simulink model "GreenHydrogenMicrogrid"  (R2026a)
settings: Solver=FixedStepAuto  StopTime=24*3600*7.5  FixedStep=Ts  MaxStep=0.1  AbsTol=1e-3
PreLoadFcn:
  | GreenHydrogenMicrogridData;
undefined symbols (not defined in the file): Battery, DiscIntNeverNeededParam, Electrolyzer, Operation_Ref, Plate, R_h2, Tank, Ts
libraries: fl_lib x35, nesl_utility x15, ee_lib x4, simulink x3, batteryecm_lib x1
(part 3 of 3)

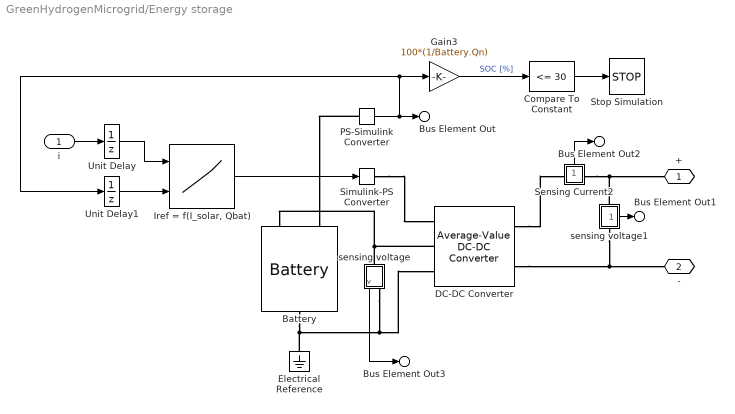
== system GreenHydrogenMicrogrid/Energy storage ==
  i : Inport
  Battery : batteryecm_lib/Battery  Vnom=Battery.Un V  prm_dir=1  R1_dis=2 Ohm  R1_ch=2 Ohm  R1=Battery.Rs Ohm  prm_AH=2  AH=Battery.Qn hr*A  V1=Battery.U1 V  AH1=Battery.Q1 hr*A  prm_R2=1  R2=2000 Ohm  Tmeas=298.15 K  charge_measurement_port=simscape.enum.battery.enable.yes  prm_dyn=1  Rp1=0.005 Ohm  tau1=30 s  Rp2=0.005 Ohm  tau2=30 s  Rp3=0.005 Ohm  tau3=30 s  Rp4=0.005 Ohm  tau4=30 s  Rp5=0.005 Ohm  tau5=30 s  prm_fade=1  N_fade=100  AH_fade=45 hr*A  R1_fade=2.02 Ohm  R1_ch_fade=2.02 Ohm  V1_fade=10.35 V  prm_age=1  prm_age_OCV=1  OCV_age=0.9  SOC_age=60  Tmeas_age=298.15 K  delta_time_age_vec=[0] d  temperature_age_vec=[273] K  OCV_scaling_age=2.2134e6  OCV_offset_age=1.632e6  temp_exp_age=0.515833569 V  t_exp_age=0.75  Vnom_T2=12 V  R1_T2=2.2 Ohm  R1_T2_dis=2.2 Ohm  R1_T2_ch=2.2 Ohm  V1_T2=11.4 V  R2_T2=2200 Ohm  Rp1_T2=0.005 Ohm  tau1_T2=30 s  Rp2_T2=0.005 Ohm  tau2_T2=30 s  Rp3_T2=0.005 Ohm  tau3_T2=30 s  Rp4_T2=0.005 Ohm  tau4_T2=30 s  Rp5_T2=0.005 Ohm  tau5_T2=30 s  Tmeas2=273.15 K  thermal_port=simscape.enum.thermaleffects.omit  thermal_mass=30000 J/K  i_specify=off  i_priority=None  i=0 A  i_nominal_specify=off  i_nominal_value=1  i_nominal_unit=A  v_specify=off  v_priority=High  v=120 V  v_nominal_specify=off  v_nominal_value=1  v_nominal_unit=V  charge_specify=on  charge_priority=High  charge=Battery.Qinit hr*A  charge_nominal_specify=off  charge_nominal_value=1  charge_nominal_unit=A*hr  num_cycles_specify=off  num_cycles_priority=High  num_cycles=0  num_cycles_nominal_specify=off  num_cycles_nominal_value=1  num_cycles_nominal_unit=1  temperature_specify=off  temperature_priority=High  temperature=298.15 K  temperature_nominal_specify=off  temperature_nominal_value=1  temperature_nominal_unit=K
      settings: LogSimulationData=on
  Compare To Constant : simulink/Logic and Bit Operations/Compare To Constant  relop=<=  const=30  OutDataTypeStr=boolean
  DC-DC Converter : ee_lib/Semiconductors & Converters/Converters/Average-Value DC-DC Converter  implementation_option=ee.enum.converters.implementation.behavioral  converter_type=ee.enum.converters.dcdctype.buck  control_option=ee.enum.converters.controlinput.current  efficiency_option=ee.enum.converters.efficiency.tabulated  efficiency_fixed=100  i_vec=Converter.Iout A  efficiency_vec=Converter.Efficiency  Lf=1e-6 H  Rl=0 Ohm  Cf=1e-7 F  Rc=1e-6 Ohm  iL_specify=off  iL_priority=High  iL=0 A  iL_nominal_specify=off  iL_nominal_value=1  iL_nominal_unit=A  vc_specify=off  vc_priority=High  vc=0 V  vc_nominal_specify=off  vc_nominal_value=1  vc_nominal_unit=V
      settings: LogSimulationData=on
  Electrical Reference : fl_lib/Electrical/Electrical Elements/Electrical Reference
  Gain3 : Gain  Gain=100*(1/Battery.Qn)
  "Iref = f(I_solar, Qbat)" : Lookup_n-D  BreakpointsForDimension1=Operation_Ref.Isolar  BreakpointsForDimension2=[0 0.5 0.875 1]*Battery.Qn  Table=[0*Operation_Ref.Ie;0.25*Operation_Ref.Ie;0.75*Operation_Ref.Ie;Operation_Ref.Ie]'  InternalRulePriority=Speed  RndMeth=Simplest
      settings: InputPortMap=u0,u1
  PS-Simulink Converter : nesl_utility/PS-Simulink Converter  PhysicalDomain=network_engine_domain  SubClassName=ps_output  LeftPortType=input  RightPortType=output  PseudoPeriodic=off  Frequencies=[]  VectorFormat=1-D array  Unit=A*hr  AffineConversion=off
  Sensing Current2 : Subsystem
      settings: PortSchema="{\"entries\":[{\"content\":{\"sides\":[{\"content\":{\"connectorIds\":[\"LConn1\"]},\"type\":\"ConnectorPlacement.EquallySpacedRectSide\",\"uuid\":\"e3c1304f-b602-4c8c-83ae-2fd3882be16e\"},{\"content\":{\"connectorIds\":[\"RConn1\"],\"side\":\"RIGHT\"},\"type\":\"ConnectorPlacement.EquallySpacedRectSide\",\"uuid\":\"8d7546a0-f580-4754-b3ac-0546585847f9\"},{\"content\":{\"connectorIds\":[\"Out1\"],\"side\":\"TOP\"},\"type\":\"ConnectorPlacement.EquallySpacedRectSide\",\"uuid\":\"be7a685a-381b-4438-acf4-f99982fa8e59\"}]},\"type\":\"ConnectorPlacement.EquallySpacedConnector\",\"uuid\":\"e35d636b-ea96-4c19-a517-3c12fcbe0b84\"}],\"packageUris\":[\"http://schema.mathworks.com/mf0/Connector/R2020b\"],\"version\":\"1.0\"}"
      mask Display: disp('i')
  Simulink-PS Converter : nesl_utility/Simulink-PS Converter  PhysicalDomain=network_engine_domain  SubClassName=ps_input  LeftPortType=input  RightPortType=output  PseudoPeriodic=off  Frequencies=[]  NoiseDistribution=none  NoiseParameters=[]  Unit=1  AffineConversion=off  FilteringAndDerivatives=provide  SimscapeFilterOrder=1  InputFilterTimeConstant=0.001  UdotUserProvided=0
  Stop Simulation : Stop
  Unit Delay : UnitDelay  SampleTime=-1
  Unit Delay1 : UnitDelay  InitialCondition=Battery.Qinit  SampleTime=-1
  sensing voltage : Subsystem
      mask Display: disp('v')
  sensing voltage1 : Subsystem
      settings: PortSchema="{\"entries\":[{\"content\":{\"sides\":[{\"content\":{\"connectorIds\":[\"LConn1\"]},\"type\":\"ConnectorPlacement.EquallySpacedRectSide\",\"uuid\":\"e3c1304f-b602-4c8c-83ae-2fd3882be16e\"},{\"content\":{\"connectorIds\":[\"RConn1\"],\"side\":\"RIGHT\"},\"type\":\"ConnectorPlacement.EquallySpacedRectSide\",\"uuid\":\"8d7546a0-f580-4754-b3ac-0546585847f9\"},{\"content\":{\"connectorIds\":[],\"side\":\"TOP\"},\"type\":\"ConnectorPlacement.EquallySpacedRectSide\",\"uuid\":\"be7a685a-381b-4438-acf4-f99982fa8e59\"},{\"content\":{\"connectorIds\":[\"Out1\"],\"side\":\"BOTTOM\"},\"type\":\"ConnectorPlacement.EquallySpacedRectSide\",\"uuid\":\"ccbd8d83-052f-4575-9126-5f77f7214aaa\"}]},\"type\":\"ConnectorPlacement.EquallySpacedConnector\",\"uuid\":\"e35d636b-ea96-4c19-a517-3c12fcbe0b84\"}],\"packageUris\":[\"http://schema.mathworks.com/mf0/Connector/R2020b\"],\"version\":\"1.0\"}"
      mask Display: disp('v')
  + : PMIOPort  Side=Left
  - : PMIOPort  Port=2  Side=Left
  Bus Element Out : Outport  PortName=visStorage  Element=Qbat
  Bus Element Out1 : Outport  PortName=visStorage  Element=v
  Bus Element Out2 : Outport  PortName=visStorage  Element=i
  Bus Element Out3 : Outport  PortName=visStorage  Element=vBatt
  wires:
  Unit Delay/1 -> "Iref = f(I_solar, Qbat)"/1
  i/1 -> Unit Delay/1
  PS-Simulink Converter/1 -> Bus Element Out/1, Gain3/1, Unit Delay1/1
  Unit Delay1/1 -> "Iref = f(I_solar, Qbat)"/2
  "Iref = f(I_solar, Qbat)"/1 -> Simulink-PS Converter/1
  sensing voltage1/1(Vstorage) -> Bus Element Out1/1
  Sensing Current2/1(Istorage) -> Bus Element Out2/1
  sensing voltage/1(v) -> Bus Element Out3/1
  Gain3/1 -> Compare To Constant/1  "SOC [%]"
  Compare To Constant/1 -> Stop Simulation/1
  connections:
  sensing voltage1/RConn1 -- -/RConn1 -- DC-DC Converter/RConn2
  Sensing Current2/RConn1 -- +/RConn1 -- sensing voltage1/LConn1
  DC-DC Converter/LConn2 -- Battery/LConn1 -- sensing voltage/LConn1
  DC-DC Converter/RConn1 -- Sensing Current2/LConn1
  Battery/RConn1 -- Electrical Reference/LConn1 -- sensing voltage/RConn1 -- DC-DC Converter/LConn3
  Simulink-PS Converter/RConn1 -- DC-DC Converter/LConn1
  PS-Simulink Converter/LConn1 -- Battery/LConn2

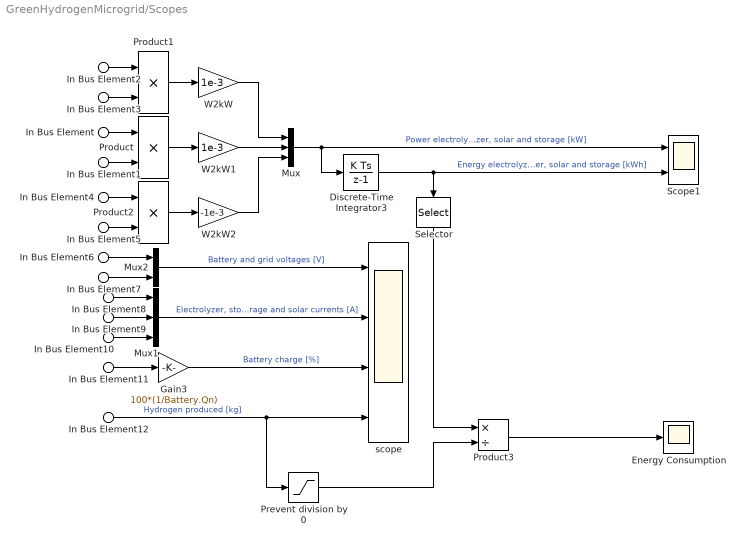
== system GreenHydrogenMicrogrid/Scopes ==
  In Bus Element2 : Inport  PortName=visElectrolyzer  Element=v
  In Bus Element3 : Inport  PortName=visElectrolyzer  Element=i
  In Bus Element8 : Inport  PortName=visElectrolyzer  Element=i
  In Bus Element12 : Inport  PortName=visElectrolyzer  Element=mH2
  In Bus Element : Inport  Port=2  PortName=visSolar  Element=v
  In Bus Element1 : Inport  Port=2  PortName=visSolar  Element=i
  In Bus Element10 : Inport  Port=2  PortName=visSolar  Element=i
  In Bus Element4 : Inport  Port=3  PortName=visStorage  Element=v
  In Bus Element7 : Inport  Port=3  PortName=visStorage  Element=v
  In Bus Element5 : Inport  Port=3  PortName=visStorage  Element=i
  In Bus Element9 : Inport  Port=3  PortName=visStorage  Element=i
  In Bus Element6 : Inport  Port=3  PortName=visStorage  Element=vBatt
  In Bus Element11 : Inport  Port=3  PortName=visStorage  Element=Qbat
  Discrete-Time Integrator3 : DiscreteIntegrator  gainval=1/3600  SampleTime=-1  ICPrevOutput=DiscIntNeverNeededParam  ICPrevScaledInput=DiscIntNeverNeededParam
  Energy Consumption : Scope
      settings: AttributesFormatString=[kWh / kg H2]  Title=Energy consumption [kWh / kgH2]  ActiveDisplayYMinimum=-8.1004  ActiveDisplayYMaximum=72.90356
  Gain3 : Gain  Gain=100*(1/Battery.Qn)
  Mux : Mux  Inputs=3
  Mux1 : Mux  Inputs=3
  Mux2 : Mux  Inputs=2
  Prevent division by 0 : Saturate  UpperLimit=inf  LowerLimit=1e-4
  Product : Product
  Product1 : Product
  Product2 : Product
  Product3 : Product  Inputs=*/
  Scope1 : Scope  NumInputPorts=2
      settings: ActiveDisplayYMinimum=-52.76446  ActiveDisplayYMaximum=231.1683
      settings: AttributesFormatString=|
      | Power
      | Energy
  Selector : Selector  InputPortWidth=3  IndexOptions=Index vector (dialog)  Indices=1  OutputSizes=1
  W2kW : Gain  Gain=1e-3
  W2kW1 : Gain  Gain=1e-3
  W2kW2 : Gain  Gain=-1e-3
  scope : Scope  NumInputPorts=4
      settings: ActiveDisplayYMinimum=211.75861  ActiveDisplayYMaximum=247.26216
      settings: AttributesFormatString=|
      | V - I
      | Charge [%]
      | H2 [kg]
  wires:
  In Bus Element1/1 -> Product/2
  In Bus Element/1 -> Product/1
  Product/1 -> W2kW1/1
  Product1/1 -> W2kW/1
  In Bus Element2/1 -> Product1/1
  In Bus Element3/1 -> Product1/2
  W2kW2/1 -> Mux/3
  Product2/1 -> W2kW2/1
  In Bus Element4/1 -> Product2/1
  In Bus Element5/1 -> Product2/2
  W2kW/1 -> Mux/1
  W2kW1/1 -> Mux/2
  Mux/1 -> Scope1/1, Discrete-Time Integrator3/1  "Power electrolyzer, solar and storage [kW]"
  Gain3/1 -> scope/3  "Battery charge [%]"
  Mux1/1 -> scope/2  "Electrolyzer, storage and solar currents [A]"
  In Bus Element12/1 -> scope/4, Prevent division by 0/1  "Hydrogen produced [kg]"
  In Bus Element6/1 -> Mux2/1
  In Bus Element7/1 -> Mux2/2
  Mux2/1 -> scope/1  "Battery and grid voltages [V]"
  In Bus Element10/1 -> Mux1/3
  In Bus Element9/1 -> Mux1/2
  Discrete-Time Integrator3/1 -> Scope1/2, Selector/1  "Energy electrolyzer, solar and storage [kWh]"
  In Bus Element11/1 -> Gain3/1
  In Bus Element8/1 -> Mux1/1
  Selector/1 -> Product3/1
  Product3/1 -> Energy Consumption/1
  Prevent division by 0/1 -> Product3/2

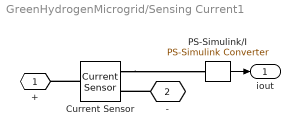
== system GreenHydrogenMicrogrid/Sensing Current1 ==
  Current Sensor : fl_lib/Electrical/Electrical Sensors/Current Sensor
  PS-Simulink/I : nesl_utility/PS-Simulink Converter  PhysicalDomain=network_engine_domain  SubClassName=ps_output  LeftPortType=input  RightPortType=output  PseudoPeriodic=off  Frequencies=[]  VectorFormat=1-D array  Unit=1  AffineConversion=off
  + : PMIOPort  Side=Left
  - : PMIOPort  Port=2  Side=Right
  iout : Outport
  wires:
  PS-Simulink/I/1 -> iout/1
  connections:
  Current Sensor/RConn1 -- PS-Simulink/I/LConn1
  Current Sensor/LConn1 -- +/RConn1
  -/RConn1 -- Current Sensor/RConn2

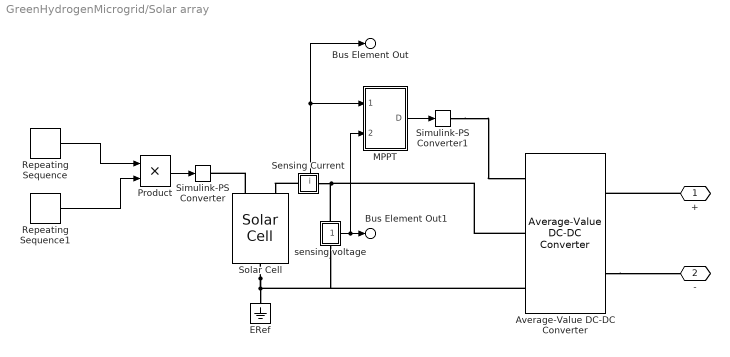
== system GreenHydrogenMicrogrid/Solar array ==
  Average-Value DC-DC Converter : ee_lib/Semiconductors & Converters/Converters/Average-Value DC-DC Converter  implementation_option=ee.enum.converters.implementation.behavioral  converter_type=ee.enum.converters.dcdctype.buckboost  control_option=ee.enum.converters.controlinput.dutycycle  efficiency_option=ee.enum.converters.efficiency.constant  efficiency_fixed=95  i_vec=[0, 2, 5] A  efficiency_vec=[90, 95, 98]  Lf=1e-6 H  Rl=0 Ohm  Cf=1e-7 F  Rc=1e-6 Ohm  iL_specify=off  iL_priority=High  iL=0 A  iL_nominal_specify=off  iL_nominal_value=1  iL_nominal_unit=A  vc_specify=off  vc_priority=High  vc=0 V  vc_nominal_specify=off  vc_nominal_value=1  vc_nominal_unit=V
  ERef : fl_lib/Electrical/Electrical Elements/Electrical Reference
  MPPT : Subsystem
  Product : Product
  Repeating Sequence : simulink/Sources/Repeating Sequence  rep_seq_t=t_solar_profile  rep_seq_y=solar_profile
  Repeating Sequence1 : simulink/Sources/Repeating Sequence  rep_seq_t=[0 1 1.1 2 2.1 3]*(3600*24)  rep_seq_y=[0.8 0.8 1 1 0.9 0.9]
  Sensing Current : Subsystem
      settings: PortSchema="{\"entries\":[{\"content\":{\"sides\":[{\"content\":{\"connectorIds\":[\"LConn1\"]},\"type\":\"ConnectorPlacement.EquallySpacedRectSide\",\"uuid\":\"e3c1304f-b602-4c8c-83ae-2fd3882be16e\"},{\"content\":{\"connectorIds\":[\"RConn1\"],\"side\":\"RIGHT\"},\"type\":\"ConnectorPlacement.EquallySpacedRectSide\",\"uuid\":\"8d7546a0-f580-4754-b3ac-0546585847f9\"},{\"content\":{\"connectorIds\":[\"Out1\"],\"side\":\"TOP\"},\"type\":\"ConnectorPlacement.EquallySpacedRectSide\",\"uuid\":\"be7a685a-381b-4438-acf4-f99982fa8e59\"}]},\"type\":\"ConnectorPlacement.EquallySpacedConnector\",\"uuid\":\"e35d636b-ea96-4c19-a517-3c12fcbe0b84\"}],\"packageUris\":[\"http://schema.mathworks.com/mf0/Connector/R2020b\"],\"version\":\"1.0\"}"
      mask Display: disp('i')
  Simulink-PS Converter : nesl_utility/Simulink-PS Converter  PhysicalDomain=network_engine_domain  SubClassName=ps_input  LeftPortType=input  RightPortType=output  PseudoPeriodic=off  Frequencies=[]  NoiseDistribution=none  NoiseParameters=[]  Unit=1  AffineConversion=off  FilteringAndDerivatives=provide  SimscapeFilterOrder=1  InputFilterTimeConstant=0.001  UdotUserProvided=0
  Simulink-PS Converter1 : nesl_utility/Simulink-PS Converter  PhysicalDomain=network_engine_domain  SubClassName=ps_input  LeftPortType=input  RightPortType=output  PseudoPeriodic=off  Frequencies=[]  NoiseDistribution=none  NoiseParameters=[]  Unit=1  AffineConversion=off  FilteringAndDerivatives=provide  SimscapeFilterOrder=1  InputFilterTimeConstant=0.001  UdotUserProvided=0
  Solar Cell : ee_lib/Sources/Solar Cell  prm=3  Isc=3.8 A  Voc=0.586 V  Is=3.15e-07 A  Is2=0 A  Iph=3.80 A  Ir0=1000 W/m^2  ec=1.4  N2=2  Rs=0.00042 Ohm  Rp=10.1 Ohm  N_series=700  N_parallel=1  TIPH1=0.000805 1/K  EG=1.14 eV  TXIS1=3.38  TXIS2=3  TRS1=0  TRP1=0  Tmeas=25 degC  TFIXED=temperature degC  thermal_mass=100 J/K  initial_temperature=25 degC
      settings: LogSimulationData=on
  sensing voltage : Subsystem
      settings: PortSchema="{\"entries\":[{\"content\":{\"sides\":[{\"content\":{\"connectorIds\":[\"LConn1\"]},\"type\":\"ConnectorPlacement.EquallySpacedRectSide\",\"uuid\":\"e3c1304f-b602-4c8c-83ae-2fd3882be16e\"},{\"content\":{\"connectorIds\":[\"RConn1\"],\"side\":\"RIGHT\"},\"type\":\"ConnectorPlacement.EquallySpacedRectSide\",\"uuid\":\"8d7546a0-f580-4754-b3ac-0546585847f9\"},{\"content\":{\"connectorIds\":[],\"side\":\"TOP\"},\"type\":\"ConnectorPlacement.EquallySpacedRectSide\",\"uuid\":\"be7a685a-381b-4438-acf4-f99982fa8e59\"},{\"content\":{\"connectorIds\":[\"Out1\"],\"side\":\"BOTTOM\"},\"type\":\"ConnectorPlacement.EquallySpacedRectSide\",\"uuid\":\"241c1147-3d2c-4214-b502-61497d53680a\"}]},\"type\":\"ConnectorPlacement.EquallySpacedConnector\",\"uuid\":\"e35d636b-ea96-4c19-a517-3c12fcbe0b84\"}],\"packageUris\":[\"http://schema.mathworks.com/mf0/Connector/R2020b\"],\"version\":\"1.0\"}"
      mask Display: disp('v')
  + : PMIOPort  Side=Right
  - : PMIOPort  Port=2  Side=Right
  Bus Element Out : Outport  PortName=visSolar  Element=i
  Bus Element Out1 : Outport  PortName=visSolar  Element=v
  wires:
  Product/1 -> Simulink-PS Converter/1
  Repeating Sequence/1 -> Product/1
  Repeating Sequence1/1 -> Product/2
  sensing voltage/1(v) -> Bus Element Out1/1, MPPT/2(Vsolar)
  MPPT/1(D) -> Simulink-PS Converter1/1
  Sensing Current/1(i) -> MPPT/1(Isolar), Bus Element Out/1
  connections:
  Sensing Current/LConn1 -- Solar Cell/LConn2
  Sensing Current/RConn1 -- Average-Value DC-DC Converter/LConn2 -- sensing voltage/LConn1
  Solar Cell/RConn1 -- sensing voltage/RConn1 -- Average-Value DC-DC Converter/LConn3 -- ERef/LConn1
  Average-Value DC-DC Converter/RConn2 -- -/RConn1
  Solar Cell/LConn1 -- Simulink-PS Converter/RConn1
  Simulink-PS Converter1/RConn1 -- Average-Value DC-DC Converter/LConn1
  +/RConn1 -- Average-Value DC-DC Converter/RConn1

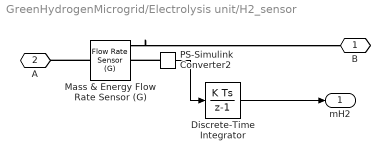
== system GreenHydrogenMicrogrid/Electrolysis unit/H2_sensor ==
  Discrete-Time Integrator : DiscreteIntegrator  gainval=1/3600  SampleTime=Ts  ICPrevOutput=DiscIntNeverNeededParam  ICPrevScaledInput=DiscIntNeverNeededParam
  Mass & Energy Flow Rate Sensor (G) : fl_lib/Gas/Sensors/Flow Rate Sensor (G)  mass_flow_measure=true  volumetric_flow_measure=false  volumetric_flow_conditions=foundation.enum.volumetric_flow_conditions.actual  p_std=0.101325 MPa  T_std=20 degC  energy_flow_measure=true
  PS-Simulink Converter2 : nesl_utility/PS-Simulink Converter  PhysicalDomain=network_engine_domain  SubClassName=ps_output  LeftPortType=input  RightPortType=output  PseudoPeriodic=off  Frequencies=[]  VectorFormat=1-D array  Unit=kg/hr  AffineConversion=off
  B : PMIOPort  Side=Left
  A : PMIOPort  Port=2  Side=Right
  mH2 : Outport
  wires:
  PS-Simulink Converter2/1 -> Discrete-Time Integrator/1
  Discrete-Time Integrator/1 -> mH2/1
  connections:
  Mass & Energy Flow Rate Sensor (G)/LConn1 -- A/RConn1
  Mass & Energy Flow Rate Sensor (G)/RConn1 -- B/RConn1
  PS-Simulink Converter2/LConn1 -- Mass & Energy Flow Rate Sensor (G)/RConn2

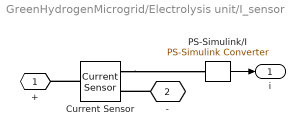
== system GreenHydrogenMicrogrid/Electrolysis unit/I_sensor ==
  Current Sensor : fl_lib/Electrical/Electrical Sensors/Current Sensor
  PS-Simulink/I : nesl_utility/PS-Simulink Converter  PhysicalDomain=network_engine_domain  SubClassName=ps_output  LeftPortType=input  RightPortType=output  PseudoPeriodic=off  Frequencies=[]  VectorFormat=1-D array  Unit=1  AffineConversion=off
  + : PMIOPort  Side=Left
  - : PMIOPort  Port=2  Side=Right
  i : Outport
  wires:
  PS-Simulink/I/1 -> i/1
  connections:
  -/RConn1 -- Current Sensor/RConn2
  Current Sensor/LConn1 -- +/RConn1
  Current Sensor/RConn1 -- PS-Simulink/I/LConn1

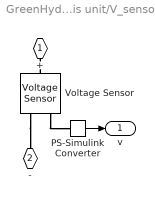
== system GreenHydrogenMicrogrid/Electrolysis unit/V_sensor ==
  PS-Simulink Converter : nesl_utility/PS-Simulink Converter  PhysicalDomain=network_engine_domain  SubClassName=ps_output  LeftPortType=input  RightPortType=output  PseudoPeriodic=off  Frequencies=[]  VectorFormat=1-D array  Unit=inherit  AffineConversion=off
  Voltage Sensor : fl_lib/Electrical/Electrical Sensors/Voltage Sensor
  + : PMIOPort  Side=Left
  - : PMIOPort  Port=2  Side=Right
  v : Outport
  wires:
  PS-Simulink Converter/1 -> v/1
  connections:
  Voltage Sensor/LConn1 -- +/RConn1
  Voltage Sensor/RConn2 -- -/RConn1
  Voltage Sensor/RConn1 -- PS-Simulink Converter/LConn1

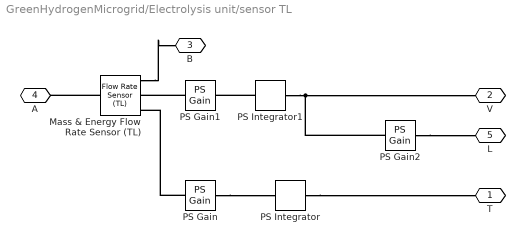
== system GreenHydrogenMicrogrid/Electrolysis unit/sensor TL ==
  Mass & Energy Flow Rate Sensor (TL) : fl_lib/Thermal Liquid/Sensors/Flow Rate Sensor (TL)  mass_flow_measure=true  volumetric_flow_measure=false  energy_flow_measure=true
  PS Gain : fl_lib/Physical Signals/Functions/PS Gain  gain=0.6/1e6 K/(W*s)
  PS Gain1 : fl_lib/Physical Signals/Functions/PS Gain  gain=1/999.84 m^3/(kg)
  PS Gain2 : fl_lib/Physical Signals/Functions/PS Gain  gain=1/(Tank.Area*1e-4) 1/m^2
  PS Integrator : fl_lib/Physical Signals/Linear Operators/PS Integrator  reset_method=foundation.enum.IntegratorResetSpec.None  initial_condition_spec=foundation.enum.IntegratorICSpec.Internal  saturation_spec=foundation.enum.IntegratorSaturationSpec.None  saturation_source_spec=foundation.enum.IntegratorSaturationSourceSpec.Internal  x0=293.15 K  xu=inf s  xl=-inf s
  PS Integrator1 : fl_lib/Physical Signals/Linear Operators/PS Integrator  reset_method=foundation.enum.IntegratorResetSpec.None  initial_condition_spec=foundation.enum.IntegratorICSpec.Internal  saturation_spec=foundation.enum.IntegratorSaturationSpec.None  saturation_source_spec=foundation.enum.IntegratorSaturationSourceSpec.Internal  x0=1.5 m^3  xu=inf s  xl=-inf s
  T : PMIOPort  Side=Left
  V : PMIOPort  Port=2  Side=Left
  B : PMIOPort  Port=3  Side=Right
  A : PMIOPort  Port=4  Side=Right
  L : PMIOPort  Port=5  Side=Right
  connections:
  Mass & Energy Flow Rate Sensor (TL)/RConn1 -- B/RConn1
  Mass & Energy Flow Rate Sensor (TL)/LConn1 -- A/RConn1
  PS Gain1/LConn1 -- Mass & Energy Flow Rate Sensor (TL)/RConn2
  PS Gain/LConn1 -- Mass & Energy Flow Rate Sensor (TL)/RConn3
  PS Gain2/LConn1 -- PS Integrator1/RConn1 -- V/RConn1
  PS Integrator1/LConn1 -- PS Gain1/RConn1
  PS Gain2/RConn1 -- L/RConn1
  PS Gain/RConn1 -- PS Integrator/LConn1
  PS Integrator/RConn1 -- T/RConn1

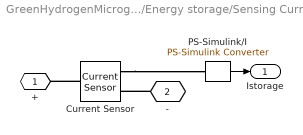
== system GreenHydrogenMicrogrid/Energy storage/Sensing Current2 ==
  Current Sensor : fl_lib/Electrical/Electrical Sensors/Current Sensor
  PS-Simulink/I : nesl_utility/PS-Simulink Converter  PhysicalDomain=network_engine_domain  SubClassName=ps_output  LeftPortType=input  RightPortType=output  PseudoPeriodic=off  Frequencies=[]  VectorFormat=1-D array  Unit=1  AffineConversion=off
  + : PMIOPort  Side=Left
  - : PMIOPort  Port=2  Side=Right
  Istorage : Outport
  wires:
  PS-Simulink/I/1 -> Istorage/1
  connections:
  Current Sensor/RConn1 -- PS-Simulink/I/LConn1
  Current Sensor/LConn1 -- +/RConn1
  -/RConn1 -- Current Sensor/RConn2

== system GreenHydrogenMicrogrid/Energy storage/sensing voltage ==
  PS-Simulink Converter : nesl_utility/PS-Simulink Converter  PhysicalDomain=network_engine_domain  SubClassName=ps_output  LeftPortType=input  RightPortType=output  PseudoPeriodic=off  Frequencies=[]  VectorFormat=1-D array  Unit=inherit  AffineConversion=off
  Voltage Sensor : fl_lib/Electrical/Electrical Sensors/Voltage Sensor
  + : PMIOPort  Side=Left
  - : PMIOPort  Port=2  Side=Right
  v : Outport
  wires:
  PS-Simulink Converter/1 -> v/1
  connections:
  Voltage Sensor/LConn1 -- +/RConn1
  Voltage Sensor/RConn2 -- -/RConn1
  Voltage Sensor/RConn1 -- PS-Simulink Converter/LConn1

== system GreenHydrogenMicrogrid/Energy storage/sensing voltage1 ==
  PS-Simulink Converter : nesl_utility/PS-Simulink Converter  PhysicalDomain=network_engine_domain  SubClassName=ps_output  LeftPortType=input  RightPortType=output  PseudoPeriodic=off  Frequencies=[]  VectorFormat=1-D array  Unit=inherit  AffineConversion=off
  Voltage Sensor : fl_lib/Electrical/Electrical Sensors/Voltage Sensor
  + : PMIOPort  Side=Left
  - : PMIOPort  Port=2  Side=Right
  Vstorage : Outport
  wires:
  PS-Simulink Converter/1 -> Vstorage/1
  connections:
  Voltage Sensor/LConn1 -- +/RConn1
  Voltage Sensor/RConn2 -- -/RConn1
  Voltage Sensor/RConn1 -- PS-Simulink Converter/LConn1

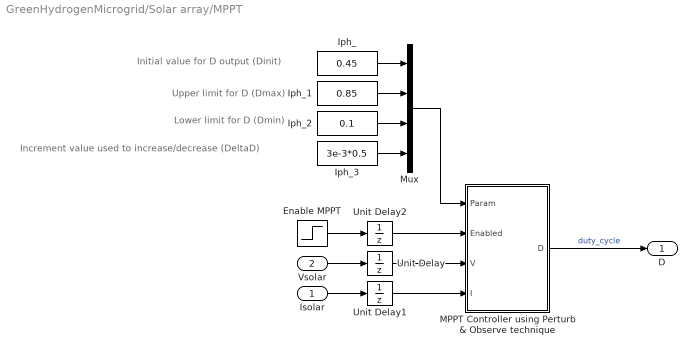
== system GreenHydrogenMicrogrid/Solar array/MPPT ==
  note: Lower limit for D (Dmin)
  note: Upper limit for D (Dmax)
  note: Increment value used to increase/decrease (DeltaD)
  note: Initial value for D output (Dinit)
  Isolar : Inport
  Vsolar : Inport  Port=2
  Enable MPPT : Step  Time=0.1  SampleTime=0
  Iph_ : Constant  Value=0.45
  Iph_1 : Constant  Value=0.85
  Iph_2 : Constant  Value=0.1
  Iph_3 : Constant  Value=3e-3*0.5
  MPPT Controller using Perturb & Observe technique : MATLAB Function  TreatAsAtomicUnit=on
  Mux : Mux
  Unit Delay : UnitDelay  SampleTime=Ts
  Unit Delay1 : UnitDelay  SampleTime=Ts
  Unit Delay2 : UnitDelay  SampleTime=Ts
  D : Outport
  wires:
  Enable MPPT/1 -> Unit Delay2/1
  Iph_3/1 -> Mux/4
  MPPT Controller using Perturb & Observe technique/1(D) -> D/1  "duty_cycle"
  Iph_2/1 -> Mux/3
  Iph_/1 -> Mux/1
  Vsolar/1 -> Unit Delay/1
  Iph_1/1 -> Mux/2
  Mux/1 -> MPPT Controller using Perturb & Observe technique/1(Param)
  Isolar/1 -> Unit Delay1/1
  Unit Delay/1 -> MPPT Controller using Perturb & Observe technique/3(V)
  Unit Delay1/1 -> MPPT Controller using Perturb & Observe technique/4(I)
  Unit Delay2/1 -> MPPT Controller using Perturb & Observe technique/2(Enabled)

== system GreenHydrogenMicrogrid/Solar array/Sensing Current ==
  Current Sensor : fl_lib/Electrical/Electrical Sensors/Current Sensor
  PS-Simulink/I : nesl_utility/PS-Simulink Converter  PhysicalDomain=network_engine_domain  SubClassName=ps_output  LeftPortType=input  RightPortType=output  PseudoPeriodic=off  Frequencies=[]  VectorFormat=1-D array  Unit=1  AffineConversion=off
  + : PMIOPort  Side=Left
  - : PMIOPort  Port=2  Side=Right
  i : Outport
  wires:
  PS-Simulink/I/1 -> i/1
  connections:
  Current Sensor/RConn1 -- PS-Simulink/I/LConn1
  Current Sensor/LConn1 -- +/RConn1
  -/RConn1 -- Current Sensor/RConn2

== system GreenHydrogenMicrogrid/Solar array/sensing voltage ==
  PS-Simulink Converter : nesl_utility/PS-Simulink Converter  PhysicalDomain=network_engine_domain  SubClassName=ps_output  LeftPortType=input  RightPortType=output  PseudoPeriodic=off  Frequencies=[]  VectorFormat=1-D array  Unit=inherit  AffineConversion=off
  Voltage Sensor : fl_lib/Electrical/Electrical Sensors/Voltage Sensor
  + : PMIOPort  Side=Left
  - : PMIOPort  Port=2  Side=Right
  v : Outport
  wires:
  PS-Simulink Converter/1 -> v/1
  connections:
  Voltage Sensor/RConn1 -- PS-Simulink Converter/LConn1
  Voltage Sensor/RConn2 -- -/RConn1
  Voltage Sensor/LConn1 -- +/RConn1

== matlab function GreenHydrogenMicrogrid/Solar array/MPPT/MPPT Controller using Perturb & Observe technique ==
  settings: updateMethod=DISCRETE
  data: Param input; D output; Enabled input; V input; I input
function D  = PandO(Param, Enabled, V, I)

% MPPT controller based on the Perturb & Observe algorithm.

% D output = Duty cycle of the boost converter (value between 0 and 1)
%
% Enabled input = 1 to enable the MPPT controller
% V input = PV array terminal voltage (V)
% I input = PV array current (A)
%
% Param input:
Dinit = Param(1);  %Initial value for D output
Dmax = Param(2);   %Maximum value for D
Dmin = Param(3);   %Minimum value for D
deltaD = Param(4); %Increment value used to increase/decrease the duty cycle D
% ( increasing D = decreasing Vref )
%  

persistent Vold Pold Dold;

if isempty(Vold)
    Vold=0;
    Pold=0;
    Dold=Dinit;
end
P= V*I;
dV= V - Vold;
dP= P - Pold;

 if dP ~= 0 && Enabled ~=0
%     if dP>1e-9  & dP<-1e-9 & Enabled ~=0
    if dP < 0
        if dV < 0
            D = Dold - deltaD;
        else
            D = Dold + deltaD;
        end
    else
        if dV < 0
            D = Dold + deltaD;
        else
            D = Dold - deltaD;
        end    
    end
 else 
     D=Dold;
end

if D >= Dmax || D<= Dmin
    D=Dold;
end

Dold=D;
Vold=V;
Pold=P;
